simulink model "projection_test"  (R2018b)
settings: Solver=VariableStepAuto  StartTime=0.0  StopTime=10.0  RelTol=1e-3
undefined symbols (not defined in the file): fswParams, simParams
libraries: dspstat3 x1, rwa_allocation_lib x1
settings Model: Creator=taylorreynolds  LastModifiedBy=Taylor

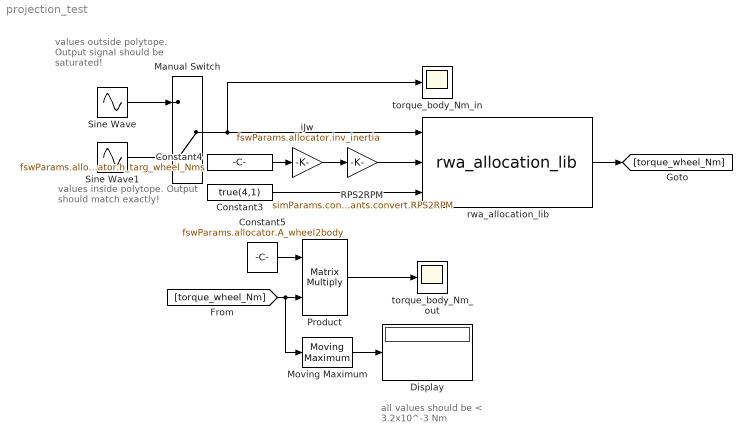
== system projection_test ==
  note: values outside polytope.
      | Output signal should be
      | saturated!
  note: values inside polytope.
      | Output should match
      | exactly!
  note: all values should be
      | < 3.2x10^-3 Nm
  Constant3 : Constant  Value=true(4,1)
  Constant4 : Constant  Value=fswParams.allocator.h_targ_wheel_Nms
  Constant5 : Constant  Value=fswParams.allocator.A_wheel2body
  Display : Display
  Manual Switch : ManualSwitch  CurrentSetting=0
  Moving Maximum : dspstat3/Moving Maximum  SpecifyWindowLength=off  WindowLength=4  SimulateUsing=Code generation
      settings: SourceProductName=DSP System Toolbox  SourceProductBaseCode=DS
  Product : Product  Multiplication=Matrix(*)
  RPS2RPM : Gain  Gain=simParams.constants.convert.RPS2RPM
  Sine Wave : Sin  Amplitude=5e-3*ones(3,1)  Bias=zeros(3,1)  Frequency=1*ones(3,1)  Phase=[0;pi;-pi/2]  SampleTime=0
  Sine Wave1 : Sin  Amplitude=2e-3*ones(3,1)  Frequency=ones(3,1)  Phase=[0;pi;-pi/2]  SampleTime=0
  iJw : Gain  Gain=fswParams.allocator.inv_inertia
  rwa_allocation_lib : rwa_allocation_lib/rwa_allocation_lib  SystemSampleTime=-1
  torque_body_Nm_in : Scope
  torque_body_Nm_out : Scope
  wires:
  Constant3/1 -> rwa_allocation_lib/3
  Constant4/1 -> iJw/1
  Constant5/1 -> Product/1
  Product/1 -> torque_body_Nm_out/1
  Manual Switch/1 -> torque_body_Nm_in/1, rwa_allocation_lib/1
  iJw/1 -> RPS2RPM/1
  RPS2RPM/1 -> rwa_allocation_lib/2
  rwa_allocation_lib/1 -> [torque_wheel_Nm]
  [torque_wheel_Nm] -> Moving Maximum/1, Product/2
  Sine Wave/1 -> Manual Switch/1
  Sine Wave1/1 -> Manual Switch/2
  Moving Maximum/1 -> Display/1
